simulink model "wall_test"  (R2017b)
settings: Solver=VariableStepAuto  StartTime=0.0  StopTime=100  RelTol=1e-7
libraries: thermochemical x1
settings Model: Creator=ferru  LastModifiedBy=fferrucc

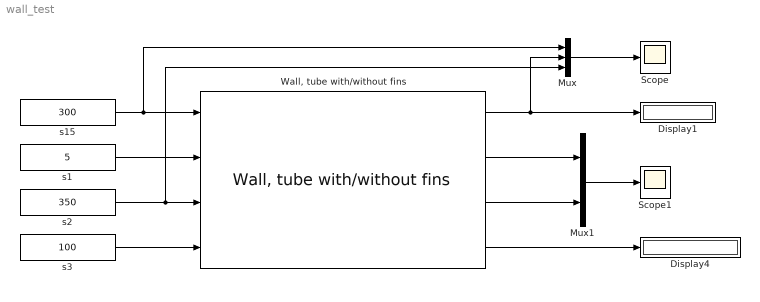
== system wall_test ==
  Display1 : Display
  Display4 : Display
  Mux : Mux  Inputs=3
  Mux1 : Mux  Inputs=2
  Scope : Scope
  Scope1 : Scope
  "Wall, tube with/without fins" : thermochemical/Walls/Wall, tube with//without fins  L_m=1  OD_mm=100  e_mm=0.1  material_tube=Aluminum 1100  cp_tube=905.9  rho_tube=2658  height_fin_mm=50  thickness_fin_mm=1  pitch_fin_mm=5  material_fin=Aluminum 1100  cp_fin=905.9  rho_fin=2658  lambda_fin=211.8  Tinit=325  mass_tube=0.08342  mass_fin=5.219  mass_total=5.3024  s_inner=0.31353  s_outer=4.2726
      settings: SourceProductName=@ Thermochemical
  s1 : Constant  Value=5
  s15 : Constant  Value=300
  s2 : Constant  Value=350
  s3 : Constant  Value=100
  wires:
  s15/1 -> Mux/1, "Wall, tube with/without fins"/1
  "Wall, tube with/without fins"/4 -> Display4/1
  s1/1 -> "Wall, tube with/without fins"/2
  s2/1 -> Mux/3, "Wall, tube with/without fins"/3
  s3/1 -> "Wall, tube with/without fins"/4
  "Wall, tube with/without fins"/1 -> Display1/1, Mux/2
  "Wall, tube with/without fins"/3 -> Mux1/2
  "Wall, tube with/without fins"/2 -> Mux1/1
  Mux/1 -> Scope/1
  Mux1/1 -> Scope1/1
